simulink model "SimulationV2"  (R2016a)
settings: Solver=ode45  StartTime=0.0  StopTime=tfin  FixedStep=0.001  RelTol=1e-09
values from neighbouring files (symbols this model uses):
  ae0 = a2(1)    [Actionneurs.m]    (also in CoefficientsActionneurs.mat = 1.33983155374)
  ae1 = a2(2)    [Actionneurs.m]    (also in CoefficientsActionneurs.mat = 355.645740125)
  ae2 = a2(3)    [Actionneurs.m]    (also in CoefficientsActionneurs.mat = 1816.89307929)
  ae3 = a2(4)    [Actionneurs.m]    (also in CoefficientsActionneurs.mat = 704384.749782)
  as0 = a3(1)    [Actionneurs.m]    (also in CoefficientsActionneurs.mat = 0.0586667067)
  as1 = a3(2)    [Actionneurs.m]    (also in CoefficientsActionneurs.mat = 22.4105523392)
  as2 = a3(3)    [Actionneurs.m]    (also in CoefficientsActionneurs.mat = 860.394175869)
  as3 = a3(4)    [Actionneurs.m]    (also in CoefficientsActionneurs.mat = 233710.908706)
  be1 = 13.029359254409743    (= 13.0293592544)    [Actionneurs.m]    (also in CoefficientsActionneurs.mat)
  g = 9.81    [bancEssaiConstantes.m]    (also in trajectoire.m = sqrt(1 + (df).^2))
  Jx = 1169e-06    (= 0.001169)    [bancEssaiConstantes.m]
  Jy = Jx    (= 0.001169)    [bancEssaiConstantes.m]
  LA = LL    (= 0.115)    [bancEssaiConstantes.m]
  LB = LL    (= 0.115)    [bancEssaiConstantes.m]
  LC = LL    (= 0.115)    [bancEssaiConstantes.m]
  mS = 0.0080    (= 0.008)    [bancEssaiConstantes.m]
  mSeff = mS+JS/rS^2    (= 0.0112)    [bancEssaiConstantes.m]
  mtot = mP + sig*mS    [bancEssaiConstantes.m]
  Pzeq = .015    (= 0.015)    [run_bancessai.m]
  RA = RR    (= 3.6)    [bancEssaiConstantes.m]
  RB = RR    (= 3.6)    [bancEssaiConstantes.m]
  RC = RR    (= 3.6)    [bancEssaiConstantes.m]
  Vmax = 16.0    (= 16)    [bancEssaiConstantes.m]
  XA = +rABC    (= 0.0952)    [bancEssaiConstantes.m]
  XB = -rABC*sind(30)    [bancEssaiConstantes.m]
  XC = -rABC*sind(30)    [bancEssaiConstantes.m]
  XD = +rDEF*sind(30)    [bancEssaiConstantes.m]
  XE = -rDEF    (= -0.08)    [bancEssaiConstantes.m]
  XF = +rDEF*sind(30)    [bancEssaiConstantes.m]
  YA = 0.0    (= 0)    [bancEssaiConstantes.m]
  YB = +rABC*cosd(30)    [bancEssaiConstantes.m]
  YC = -rABC*cosd(30)    [bancEssaiConstantes.m]
  YD = +rDEF*cosd(30)    [bancEssaiConstantes.m]
  YE = 0.0    (= 0)    [bancEssaiConstantes.m]
  YF = -rDEF*cosd(30)    [bancEssaiConstantes.m]
settings Model: Creator=delafontaine  LastModifiedBy=Jaco_
settings SolverCC: AlgebraicLoopSolver=LineSearch
settings DataIOCC: LimitDataPoints=on  SaveFormat=Array  SignalLoggingSaveFormat=ModelDataLogs
settings DebuggingCC: UnderspecifiedInitializationDetection=Classic  MergeDetectMultiDrivingBlocksExec=none  MultiTaskDSMMsg=warning  MultiTaskCondExecSysMsg=none
settings HardwareCC: ProdBitPerPointer=32  ProdLargestAtomicFloat=None  ProdIntDivRoundTo=Undefined  ProdEndianess=Unspecified  ProdWordSize=32  ProdHWDeviceType=32-bit Generic
settings ModelReferenceCC: PropagateSignalLabelsOutOfModel=off
settings ConfigComp: CovModelRefEnable=Off  CovSFcnEnable=off

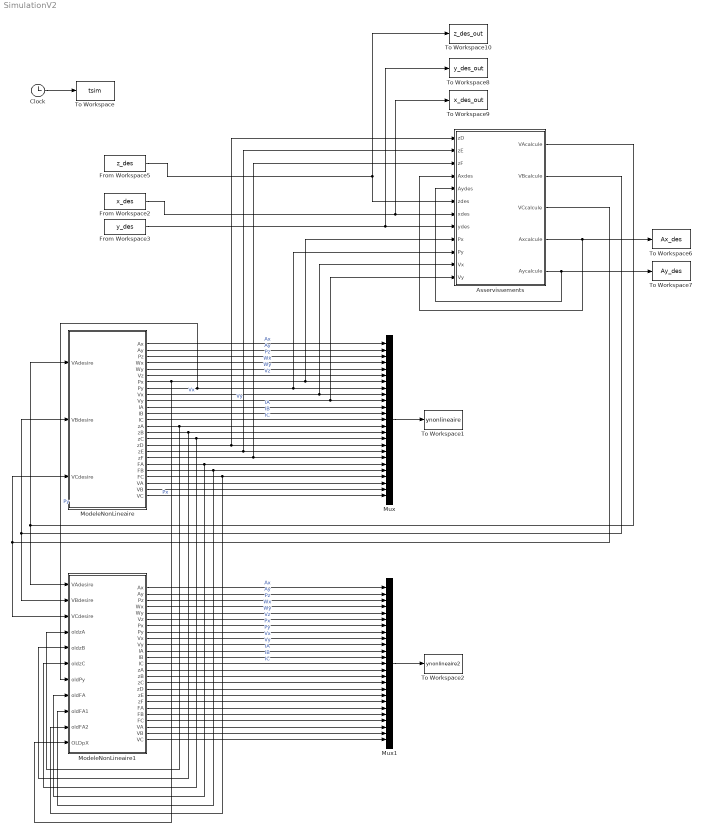
== system SimulationV2 ==
  Asservissements : Subsystem
      mask help: Simulink:masks:GenSFuncDesc_MD
      mask Help: eval('feval(''rtwprivate'',''rtwhelpview'',''rtw_sfcn_block'')');
  Clock : Clock
  From Workspace2 : FromWorkspace  VariableName=x_des  SampleTime=0  Interpolate=off  OutputAfterFinalValue=Holding final value
  From Workspace3 : FromWorkspace  VariableName=y_des  SampleTime=0  Interpolate=off  OutputAfterFinalValue=Holding final value
  From Workspace5 : FromWorkspace  VariableName=z_des  SampleTime=0  Interpolate=off  OutputAfterFinalValue=Holding final value
  ModeleNonLineaire : Subsystem
      mask help: Simulink:masks:GenSFuncDesc_MD
      mask Help: eval('feval(''rtwprivate'',''rtwhelpview'',''rtw_sfcn_block'')');
  ModeleNonLineaire1 : Subsystem
      mask help: Simulink:masks:GenSFuncDesc_MD
      mask Help: eval('feval(''rtwprivate'',''rtwhelpview'',''rtw_sfcn_block'')');
  Mux : Mux  Inputs=25
  Mux1 : Mux  Inputs=25
  To Workspace : ToWorkspace  VariableName=tsim  SampleTime=-1
  To Workspace1 : ToWorkspace  VariableName=ynonlineaire  SampleTime=-1
  To Workspace10 : ToWorkspace  VariableName=z_des_out  SampleTime=-1
  To Workspace2 : ToWorkspace  VariableName=ynonlineaire2  SampleTime=-1
  To Workspace6 : ToWorkspace  VariableName=Ax_des  SampleTime=-1
  To Workspace7 : ToWorkspace  VariableName=Ay_des  SampleTime=-1
  To Workspace8 : ToWorkspace  VariableName=y_des_out  SampleTime=-1
  To Workspace9 : ToWorkspace  VariableName=x_des_out  SampleTime=-1
  wires:
  Mux/1 -> To Workspace1/1
  Clock/1 -> To Workspace/1
  From Workspace5/1 -> Asservissements/6(zdes), To Workspace10/1
  ModeleNonLineaire/1(Ax) -> Mux/1  "Ax"
  ModeleNonLineaire/2(Ay) -> Mux/2  "Ay"
  ModeleNonLineaire/3(Pz) -> Mux/3  "Pz"
  ModeleNonLineaire/4(Wx) -> Mux/4  "Wx"
  ModeleNonLineaire/5(Wy) -> Mux/5  "Wy"
  ModeleNonLineaire/6(Vz) -> Mux/6  "Vz"
  ModeleNonLineaire/7(Px) -> ModeleNonLineaire1/11("OLDpX "), Asservissements/9(Px), Mux/7  "Px"
  ModeleNonLineaire/8(Py) -> ModeleNonLineaire1/7(oldPy), Asservissements/10(Py), Mux/8  "Py"
  ModeleNonLineaire/9(Vx) -> Asservissements/11(Vx), Mux/9  "Vx"
  ModeleNonLineaire/10(Vy) -> Asservissements/12(Vy), Mux/10  "Vy"
  ModeleNonLineaire/11(IA) -> Mux/11  "IA"
  ModeleNonLineaire/12(IB) -> Mux/12  "IB"
  ModeleNonLineaire/13(IC) -> Mux/13  "IC"
  From Workspace3/1 -> Asservissements/8(ydes), To Workspace8/1
  From Workspace2/1 -> Asservissements/7(xdes), To Workspace9/1
  ModeleNonLineaire/20(FA) -> ModeleNonLineaire1/8(oldFA), Mux/20
  ModeleNonLineaire/21(FB) -> ModeleNonLineaire1/9(oldFA1), Mux/21
  ModeleNonLineaire/22(FC) -> ModeleNonLineaire1/10(oldFA2), Mux/22
  ModeleNonLineaire/23(VA) -> Mux/23
  ModeleNonLineaire/24(VB) -> Mux/24
  ModeleNonLineaire/25(VC) -> Mux/25
  ModeleNonLineaire/17(zD) -> Asservissements/1(zD), Mux/17
  ModeleNonLineaire/18(zE) -> Asservissements/2(zE), Mux/18
  ModeleNonLineaire/19(zF) -> Asservissements/3(zF), Mux/19
  ModeleNonLineaire/14(zA) -> ModeleNonLineaire1/4(oldzA), Mux/14
  ModeleNonLineaire/15(zB) -> ModeleNonLineaire1/5(oldzB), Mux/15
  ModeleNonLineaire/16(zC) -> ModeleNonLineaire1/6(oldzC), Mux/16
  Asservissements/4(Axcalcule) -> Asservissements/4(Axdes), To Workspace6/1
  Asservissements/5(Aycalcule) -> Asservissements/5(Aydes), To Workspace7/1
  Mux1/1 -> To Workspace2/1
  ModeleNonLineaire1/1(Ax) -> Mux1/1  "Ax"
  ModeleNonLineaire1/2(Ay) -> Mux1/2  "Ay"
  ModeleNonLineaire1/3(Pz) -> Mux1/3  "Pz"
  ModeleNonLineaire1/4(Wx) -> Mux1/4  "Wx"
  ModeleNonLineaire1/5(Wy) -> Mux1/5  "Wy"
  ModeleNonLineaire1/6(Vz) -> Mux1/6  "Vz"
  ModeleNonLineaire1/7(Px) -> Mux1/7  "Px"
  ModeleNonLineaire1/8(Py) -> Mux1/8  "Py"
  ModeleNonLineaire1/9(Vx) -> Mux1/9  "Vx"
  ModeleNonLineaire1/10(Vy) -> Mux1/10  "Vy"
  ModeleNonLineaire1/11(IA) -> Mux1/11  "IA"
  ModeleNonLineaire1/12(IB) -> Mux1/12  "IB"
  ModeleNonLineaire1/13(IC) -> Mux1/13  "IC"
  ModeleNonLineaire1/20(FA) -> Mux1/20
  ModeleNonLineaire1/21(FB) -> Mux1/21
  ModeleNonLineaire1/22(FC) -> Mux1/22
  ModeleNonLineaire1/23(VA) -> Mux1/23
  ModeleNonLineaire1/24(VB) -> Mux1/24
  ModeleNonLineaire1/25(VC) -> Mux1/25
  ModeleNonLineaire1/17(zD) -> Mux1/17
  ModeleNonLineaire1/18(zE) -> Mux1/18
  ModeleNonLineaire1/19(zF) -> Mux1/19
  ModeleNonLineaire1/14(zA) -> Mux1/14
  ModeleNonLineaire1/15(zB) -> Mux1/15
  ModeleNonLineaire1/16(zC) -> Mux1/16
  Asservissements/1(VAcalcule) -> ModeleNonLineaire/1(VAdesire), ModeleNonLineaire1/1(VAdesire)
  Asservissements/2(VBcalcule) -> ModeleNonLineaire/2(VBdesire), ModeleNonLineaire1/2(VBdesire)
  Asservissements/3(VCcalcule) -> ModeleNonLineaire/3(VCdesire), ModeleNonLineaire1/3(VCdesire)

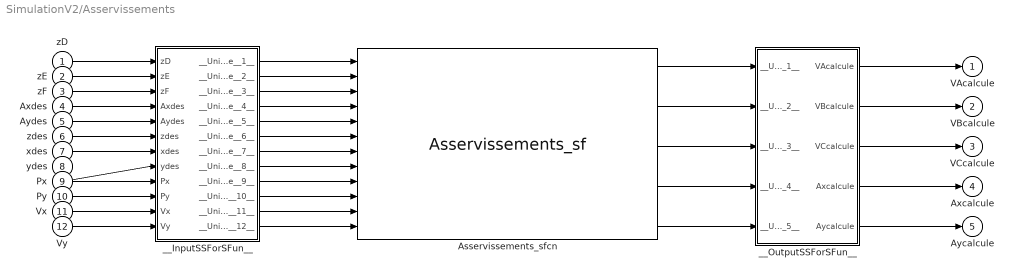
== system SimulationV2/Asservissements ==
  zD : Inport
  zE : Inport  Port=2
  zF : Inport  Port=3
  Axdes : Inport  Port=4
  Aydes : Inport  Port=5
  zdes : Inport  Port=6
  xdes : Inport  Port=7
  ydes : Inport  Port=8
  Px : Inport  Port=9
  Py : Inport  Port=10
  Vx : Inport  Port=11
  Vy : Inport  Port=12
  Asservissements_sfcn : S-Function  FunctionName=Asservissements_sf  SFunctionModules=""  SFunctionDeploymentMode=off  EnableBusSupport=off  mask{rtw_sf_name=Asservissements_sf, showVar=off}
      mask prompts: rtw_sf_name "Simulink:masks:GenSFuncName_MP"; showVar "Simulink:masks:GenSFuncShowModuleList_MP"
      mask help: Simulink:masks:GenSFuncDesc_MD
      mask init:
      | displist = '';
      | if ~strcmp(get_param(gcb, 'FunctionName'), rtw_sf_name);
      |   set_param(gcb, 'FunctionName', rtw_sf_name);
      | end
      | % Check if we are generating code
      | rtw_mode = false;
      | if strcmpi(get_param(bdroot(gcb),'SimulationStatus'),'Initializing')
      | 	rtw_mode = strcmpi(get_param(bdroot(gcb),'BuildingRTWCode'),'on') && ...
      | 		~strcmpi(get_param(bdroot(gcb),'TargetStyle'),'SimulationTarget');
      | end
      | if showVar || rtw_mode
      | 	if exist('rtwsfunc') == 2 | exist('rtwsfunc') == 6
      | 		tmplist = rtwsfunc(rtw_sf_name,gcb);
      | 		tmplist = DAStudio.message('Simulink:masks:GenSFuncListOfModules_IC', tmplist);
      | 	elseif showVar
      | 		tmplist1 = DAStudio.message('Simulink:masks:GenSFuncListOfModules_IC', '');
      |         tmplist2 = DAStudio.message('Simulink:masks:GenSFuncNotLicensed_IC');
      |         tmplist = [tmplist1 tmplist2];
      |  	end
      | end
      | if showVar
      |   displist = tmplist;
      | end
      settings: CopyFcn=|
      | if ~strcmp(get_param(gcb,'Linkstatus'),'none') && ...
      | ~strcmp(get_param(gcb,'Linkstatus'),'implicit')
      |   set_param(gcb,'LinkStatus','none');
      | end
      mask Help: eval('feval(''rtwprivate'',''rtwhelpview'',''rtw_sfcn_block'')');
      mask Display:
      | port_label('input',1,'zD');
      | port_label('input',2,'zE');
      | port_label('input',3,'zF');
      | port_label('input',4,'Axdes');
      | port_label('input',5,'Aydes');
      | port_label('input',6,'zdes');
      | port_label('input',7,'xdes');
      | port_label('input',8,'ydes');
      | port_label('input',9,'Px');
      | port_label('input',10,'Py');
      | port_label('input',11,'Vx');
      | port_label('input',12,'Vy');
      | port_label('output',1,'VAcalcule');
      | port_label('output',2,'VBcalcule');
      | port_label('output',3,'VCcalcule');
      | port_label('output',4,'Axcalcule');
      | port_label('output',5,'Aycalcule');
  __InputSSForSFun__ : Subsystem
  __OutputSSForSFun__ : Subsystem
  VAcalcule : Outport
  VBcalcule : Outport  Port=2
  VCcalcule : Outport  Port=3
  Axcalcule : Outport  Port=4
  Aycalcule : Outport  Port=5
  wires:
  zD/1 -> __InputSSForSFun__/1(zD)
  zE/1 -> __InputSSForSFun__/2(zE)
  zF/1 -> __InputSSForSFun__/3(zF)
  Axdes/1 -> __InputSSForSFun__/4(Axdes)
  Aydes/1 -> __InputSSForSFun__/5(Aydes)
  zdes/1 -> __InputSSForSFun__/6(zdes)
  xdes/1 -> __InputSSForSFun__/7(xdes)
  ydes/1 -> __InputSSForSFun__/8(ydes)
  Px/1 -> __InputSSForSFun__/9(Px)
  Py/1 -> __InputSSForSFun__/10(Py)
  Vx/1 -> __InputSSForSFun__/11(Vx)
  Vy/1 -> __InputSSForSFun__/12(Vy)
  __InputSSForSFun__/1(__UniqueOutportName__1__) -> Asservissements_sfcn/1
  __InputSSForSFun__/2(__UniqueOutportName__2__) -> Asservissements_sfcn/2
  __InputSSForSFun__/3(__UniqueOutportName__3__) -> Asservissements_sfcn/3
  __InputSSForSFun__/4(__UniqueOutportName__4__) -> Asservissements_sfcn/4
  __InputSSForSFun__/5(__UniqueOutportName__5__) -> Asservissements_sfcn/5
  __InputSSForSFun__/6(__UniqueOutportName__6__) -> Asservissements_sfcn/6
  __InputSSForSFun__/7(__UniqueOutportName__7__) -> Asservissements_sfcn/7
  __InputSSForSFun__/8(__UniqueOutportName__8__) -> Asservissements_sfcn/8
  __InputSSForSFun__/9(__UniqueOutportName__9__) -> Asservissements_sfcn/9
  __InputSSForSFun__/10(__UniqueOutportName__10__) -> Asservissements_sfcn/10
  __InputSSForSFun__/11(__UniqueOutportName__11__) -> Asservissements_sfcn/11
  __InputSSForSFun__/12(__UniqueOutportName__12__) -> Asservissements_sfcn/12
  Asservissements_sfcn/1 -> __OutputSSForSFun__/1(__UniqueInportName__1__)
  Asservissements_sfcn/2 -> __OutputSSForSFun__/2(__UniqueInportName__2__)
  Asservissements_sfcn/3 -> __OutputSSForSFun__/3(__UniqueInportName__3__)
  Asservissements_sfcn/4 -> __OutputSSForSFun__/4(__UniqueInportName__4__)
  Asservissements_sfcn/5 -> __OutputSSForSFun__/5(__UniqueInportName__5__)
  __OutputSSForSFun__/1(VAcalcule) -> VAcalcule/1
  __OutputSSForSFun__/2(VBcalcule) -> VBcalcule/1
  __OutputSSForSFun__/3(VCcalcule) -> VCcalcule/1
  __OutputSSForSFun__/4(Axcalcule) -> Axcalcule/1
  __OutputSSForSFun__/5(Aycalcule) -> Aycalcule/1

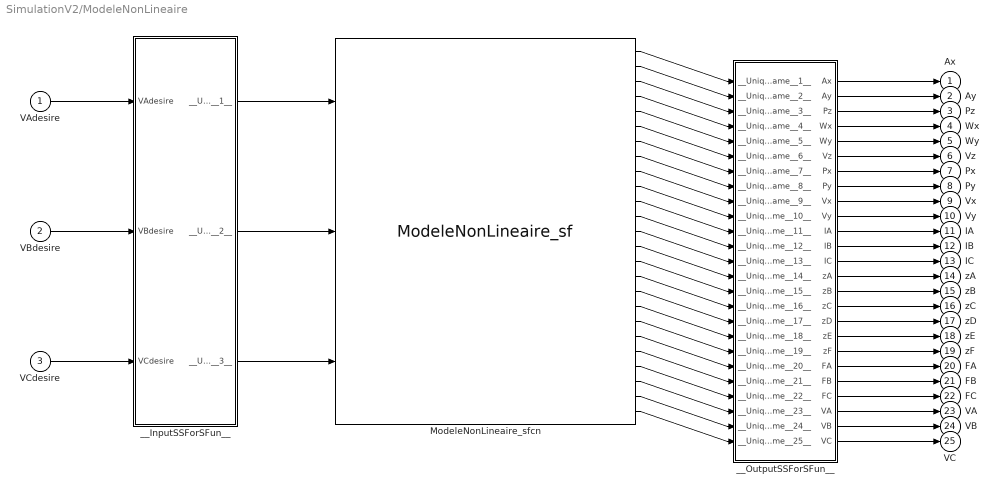
== system SimulationV2/ModeleNonLineaire ==
  VAdesire : Inport
  VBdesire : Inport  Port=2
  VCdesire : Inport  Port=3
  ModeleNonLineaire_sfcn : S-Function  FunctionName=ModeleNonLineaire_sf  SFunctionModules=""  SFunctionDeploymentMode=off  EnableBusSupport=off  mask{rtw_sf_name=ModeleNonLineaire_sf, showVar=off}
      mask prompts: rtw_sf_name "Simulink:masks:GenSFuncName_MP"; showVar "Simulink:masks:GenSFuncShowModuleList_MP"
      mask help: Simulink:masks:GenSFuncDesc_MD
      mask init: same as SimulationV2/Asservissements/Asservissements_sfcn
      settings: CopyFcn=|
      | if ~strcmp(get_param(gcb,'Linkstatus'),'none') && ...
      | ~strcmp(get_param(gcb,'Linkstatus'),'implicit')
      |   set_param(gcb,'LinkStatus','none');
      | end
      mask Help: eval('feval(''rtwprivate'',''rtwhelpview'',''rtw_sfcn_block'')');
      mask Display:
      | port_label('input',1,'VAdesire');
      | port_label('input',2,'VBdesire');
      | port_label('input',3,'VCdesire');
      | port_label('output',1,'Ax');
      | port_label('output',2,'Ay');
      | port_label('output',3,'Pz');
      | port_label('output',4,'Wx');
      | port_label('output',5,'Wy');
      | port_label('output',6,'Vz');
      | port_label('output',7,'Px');
      | port_label('output',8,'Py');
      | port_label('output',9,'Vx');
      | port_label('output',10,'Vy');
      | port_label('output',11,'IA');
      | port_label('output',12,'IB');
      | port_label('output',13,'IC');
      | port_label('output',14,'zA');
      | port_label('output',15,'zB');
      | port_label('output',16,'zC');
      | port_label('output',17,'zD');
      | port_label('output',18,'zE');
      | port_label('output',19,'zF');
      | port_label('output',20,'FA');
      | port_label('output',21,'FB');
      | port_label('output',22,'FC');
      | port_label('output',23,'VA');
      | port_label('output',24,'VB');
      | port_label('output',25,'VC');
  __InputSSForSFun__ : Subsystem
  __OutputSSForSFun__ : Subsystem
  Ax : Outport
  Ay : Outport  Port=2
  Pz : Outport  Port=3
  Wx : Outport  Port=4
  Wy : Outport  Port=5
  Vz : Outport  Port=6
  Px : Outport  Port=7
  Py : Outport  Port=8
  Vx : Outport  Port=9
  Vy : Outport  Port=10
  IA : Outport  Port=11
  IB : Outport  Port=12
  IC : Outport  Port=13
  zA : Outport  Port=14
  zB : Outport  Port=15
  zC : Outport  Port=16
  zD : Outport  Port=17
  zE : Outport  Port=18
  zF : Outport  Port=19
  FA : Outport  Port=20
  FB : Outport  Port=21
  FC : Outport  Port=22
  VA : Outport  Port=23
  VB : Outport  Port=24
  VC : Outport  Port=25
  wires:
  VAdesire/1 -> __InputSSForSFun__/1(VAdesire)
  VBdesire/1 -> __InputSSForSFun__/2(VBdesire)
  VCdesire/1 -> __InputSSForSFun__/3(VCdesire)
  __InputSSForSFun__/1(__UniqueOutportName__1__) -> ModeleNonLineaire_sfcn/1
  __InputSSForSFun__/2(__UniqueOutportName__2__) -> ModeleNonLineaire_sfcn/2
  __InputSSForSFun__/3(__UniqueOutportName__3__) -> ModeleNonLineaire_sfcn/3
  ModeleNonLineaire_sfcn/1 -> __OutputSSForSFun__/1(__UniqueInportName__1__)
  ModeleNonLineaire_sfcn/2 -> __OutputSSForSFun__/2(__UniqueInportName__2__)
  ModeleNonLineaire_sfcn/3 -> __OutputSSForSFun__/3(__UniqueInportName__3__)
  ModeleNonLineaire_sfcn/4 -> __OutputSSForSFun__/4(__UniqueInportName__4__)
  ModeleNonLineaire_sfcn/5 -> __OutputSSForSFun__/5(__UniqueInportName__5__)
  ModeleNonLineaire_sfcn/6 -> __OutputSSForSFun__/6(__UniqueInportName__6__)
  ModeleNonLineaire_sfcn/7 -> __OutputSSForSFun__/7(__UniqueInportName__7__)
  ModeleNonLineaire_sfcn/8 -> __OutputSSForSFun__/8(__UniqueInportName__8__)
  ModeleNonLineaire_sfcn/9 -> __OutputSSForSFun__/9(__UniqueInportName__9__)
  ModeleNonLineaire_sfcn/10 -> __OutputSSForSFun__/10(__UniqueInportName__10__)
  ModeleNonLineaire_sfcn/11 -> __OutputSSForSFun__/11(__UniqueInportName__11__)
  ModeleNonLineaire_sfcn/12 -> __OutputSSForSFun__/12(__UniqueInportName__12__)
  ModeleNonLineaire_sfcn/13 -> __OutputSSForSFun__/13(__UniqueInportName__13__)
  ModeleNonLineaire_sfcn/14 -> __OutputSSForSFun__/14(__UniqueInportName__14__)
  ModeleNonLineaire_sfcn/15 -> __OutputSSForSFun__/15(__UniqueInportName__15__)
  ModeleNonLineaire_sfcn/16 -> __OutputSSForSFun__/16(__UniqueInportName__16__)
  ModeleNonLineaire_sfcn/17 -> __OutputSSForSFun__/17(__UniqueInportName__17__)
  ModeleNonLineaire_sfcn/18 -> __OutputSSForSFun__/18(__UniqueInportName__18__)
  ModeleNonLineaire_sfcn/19 -> __OutputSSForSFun__/19(__UniqueInportName__19__)
  ModeleNonLineaire_sfcn/20 -> __OutputSSForSFun__/20(__UniqueInportName__20__)
  ModeleNonLineaire_sfcn/21 -> __OutputSSForSFun__/21(__UniqueInportName__21__)
  ModeleNonLineaire_sfcn/22 -> __OutputSSForSFun__/22(__UniqueInportName__22__)
  ModeleNonLineaire_sfcn/23 -> __OutputSSForSFun__/23(__UniqueInportName__23__)
  ModeleNonLineaire_sfcn/24 -> __OutputSSForSFun__/24(__UniqueInportName__24__)
  ModeleNonLineaire_sfcn/25 -> __OutputSSForSFun__/25(__UniqueInportName__25__)
  __OutputSSForSFun__/1(Ax) -> Ax/1
  __OutputSSForSFun__/2(Ay) -> Ay/1
  __OutputSSForSFun__/3(Pz) -> Pz/1
  __OutputSSForSFun__/4(Wx) -> Wx/1
  __OutputSSForSFun__/5(Wy) -> Wy/1
  __OutputSSForSFun__/6(Vz) -> Vz/1
  __OutputSSForSFun__/7(Px) -> Px/1
  __OutputSSForSFun__/8(Py) -> Py/1
  __OutputSSForSFun__/9(Vx) -> Vx/1
  __OutputSSForSFun__/10(Vy) -> Vy/1
  __OutputSSForSFun__/11(IA) -> IA/1
  __OutputSSForSFun__/12(IB) -> IB/1
  __OutputSSForSFun__/13(IC) -> IC/1
  __OutputSSForSFun__/14(zA) -> zA/1
  __OutputSSForSFun__/15(zB) -> zB/1
  __OutputSSForSFun__/16(zC) -> zC/1
  __OutputSSForSFun__/17(zD) -> zD/1
  __OutputSSForSFun__/18(zE) -> zE/1
  __OutputSSForSFun__/19(zF) -> zF/1
  __OutputSSForSFun__/20(FA) -> FA/1
  __OutputSSForSFun__/21(FB) -> FB/1
  __OutputSSForSFun__/22(FC) -> FC/1
  __OutputSSForSFun__/23(VA) -> VA/1
  __OutputSSForSFun__/24(VB) -> VB/1
  __OutputSSForSFun__/25(VC) -> VC/1

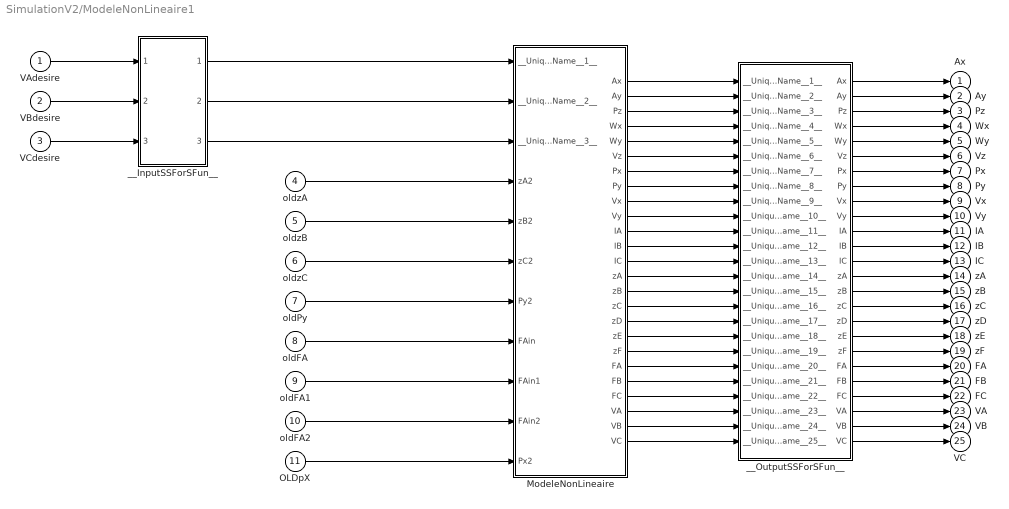
== system SimulationV2/ModeleNonLineaire1 ==
  VAdesire : Inport
  VBdesire : Inport  Port=2
  VCdesire : Inport  Port=3
  oldzA : Inport  Port=4
  oldzB : Inport  Port=5
  oldzC : Inport  Port=6
  oldPy : Inport  Port=7
  oldFA : Inport  Port=8
  oldFA1 : Inport  Port=9
  oldFA2 : Inport  Port=10
  "OLDpX " : Inport  Port=11
  ModeleNonLineaire : Subsystem
  __InputSSForSFun__ : Subsystem
  __OutputSSForSFun__ : Subsystem
  Ax : Outport
  Ay : Outport  Port=2
  Pz : Outport  Port=3
  Wx : Outport  Port=4
  Wy : Outport  Port=5
  Vz : Outport  Port=6
  Px : Outport  Port=7
  Py : Outport  Port=8
  Vx : Outport  Port=9
  Vy : Outport  Port=10
  IA : Outport  Port=11
  IB : Outport  Port=12
  IC : Outport  Port=13
  zA : Outport  Port=14
  zB : Outport  Port=15
  zC : Outport  Port=16
  zD : Outport  Port=17
  zE : Outport  Port=18
  zF : Outport  Port=19
  FA : Outport  Port=20
  FB : Outport  Port=21
  FC : Outport  Port=22
  VA : Outport  Port=23
  VB : Outport  Port=24
  VC : Outport  Port=25
  wires:
  VAdesire/1 -> __InputSSForSFun__/1(VAdesire)
  VBdesire/1 -> __InputSSForSFun__/2(VBdesire)
  VCdesire/1 -> __InputSSForSFun__/3(VCdesire)
  __InputSSForSFun__/1(__UniqueOutportName__1__) -> ModeleNonLineaire/1(__UniqueInportName__1__)
  __InputSSForSFun__/2(__UniqueOutportName__2__) -> ModeleNonLineaire/2(__UniqueInportName__2__)
  __InputSSForSFun__/3(__UniqueOutportName__3__) -> ModeleNonLineaire/3(__UniqueInportName__3__)
  __OutputSSForSFun__/1(Ax) -> Ax/1
  __OutputSSForSFun__/2(Ay) -> Ay/1
  __OutputSSForSFun__/3(Pz) -> Pz/1
  __OutputSSForSFun__/4(Wx) -> Wx/1
  __OutputSSForSFun__/5(Wy) -> Wy/1
  __OutputSSForSFun__/6(Vz) -> Vz/1
  __OutputSSForSFun__/7(Px) -> Px/1
  __OutputSSForSFun__/8(Py) -> Py/1
  __OutputSSForSFun__/9(Vx) -> Vx/1
  __OutputSSForSFun__/10(Vy) -> Vy/1
  __OutputSSForSFun__/11(IA) -> IA/1
  __OutputSSForSFun__/12(IB) -> IB/1
  __OutputSSForSFun__/13(IC) -> IC/1
  __OutputSSForSFun__/14(zA) -> zA/1
  __OutputSSForSFun__/15(zB) -> zB/1
  __OutputSSForSFun__/16(zC) -> zC/1
  __OutputSSForSFun__/17(zD) -> zD/1
  __OutputSSForSFun__/18(zE) -> zE/1
  __OutputSSForSFun__/19(zF) -> zF/1
  __OutputSSForSFun__/20(FA) -> FA/1
  __OutputSSForSFun__/21(FB) -> FB/1
  __OutputSSForSFun__/22(FC) -> FC/1
  __OutputSSForSFun__/23(VA) -> VA/1
  __OutputSSForSFun__/24(VB) -> VB/1
  __OutputSSForSFun__/25(VC) -> VC/1
  ModeleNonLineaire/23(VA) -> __OutputSSForSFun__/23(__UniqueInportName__23__)
  ModeleNonLineaire/24(VB) -> __OutputSSForSFun__/24(__UniqueInportName__24__)
  ModeleNonLineaire/25(VC) -> __OutputSSForSFun__/25(__UniqueInportName__25__)
  ModeleNonLineaire/11(IA) -> __OutputSSForSFun__/11(__UniqueInportName__11__)
  ModeleNonLineaire/12(IB) -> __OutputSSForSFun__/12(__UniqueInportName__12__)
  ModeleNonLineaire/13(IC) -> __OutputSSForSFun__/13(__UniqueInportName__13__)
  ModeleNonLineaire/20(FA) -> __OutputSSForSFun__/20(__UniqueInportName__20__)
  ModeleNonLineaire/21(FB) -> __OutputSSForSFun__/21(__UniqueInportName__21__)
  ModeleNonLineaire/22(FC) -> __OutputSSForSFun__/22(__UniqueInportName__22__)
  oldzA/1 -> ModeleNonLineaire/4(zA2)
  oldzB/1 -> ModeleNonLineaire/5(zB2)
  oldzC/1 -> ModeleNonLineaire/6(zC2)
  ModeleNonLineaire/6(Vz) -> __OutputSSForSFun__/6(__UniqueInportName__6__)
  oldPy/1 -> ModeleNonLineaire/7(Py2)
  ModeleNonLineaire/4(Wx) -> __OutputSSForSFun__/4(__UniqueInportName__4__)
  oldFA/1 -> ModeleNonLineaire/8(FAin)
  oldFA1/1 -> ModeleNonLineaire/9(FAin1)
  oldFA2/1 -> ModeleNonLineaire/10(FAin2)
  "OLDpX "/1 -> ModeleNonLineaire/11(Px2)
  ModeleNonLineaire/5(Wy) -> __OutputSSForSFun__/5(__UniqueInportName__5__)
  ModeleNonLineaire/1(Ax) -> __OutputSSForSFun__/1(__UniqueInportName__1__)
  ModeleNonLineaire/2(Ay) -> __OutputSSForSFun__/2(__UniqueInportName__2__)
  ModeleNonLineaire/14(zA) -> __OutputSSForSFun__/14(__UniqueInportName__14__)
  ModeleNonLineaire/15(zB) -> __OutputSSForSFun__/15(__UniqueInportName__15__)
  ModeleNonLineaire/16(zC) -> __OutputSSForSFun__/16(__UniqueInportName__16__)
  ModeleNonLineaire/17(zD) -> __OutputSSForSFun__/17(__UniqueInportName__17__)
  ModeleNonLineaire/18(zE) -> __OutputSSForSFun__/18(__UniqueInportName__18__)
  ModeleNonLineaire/19(zF) -> __OutputSSForSFun__/19(__UniqueInportName__19__)
  ModeleNonLineaire/3(Pz) -> __OutputSSForSFun__/3(__UniqueInportName__3__)
  ModeleNonLineaire/10(Vy) -> __OutputSSForSFun__/10(__UniqueInportName__10__)
  ModeleNonLineaire/9(Vx) -> __OutputSSForSFun__/9(__UniqueInportName__9__)
  ModeleNonLineaire/8(Py) -> __OutputSSForSFun__/8(__UniqueInportName__8__)
  ModeleNonLineaire/7(Px) -> __OutputSSForSFun__/7(__UniqueInportName__7__)

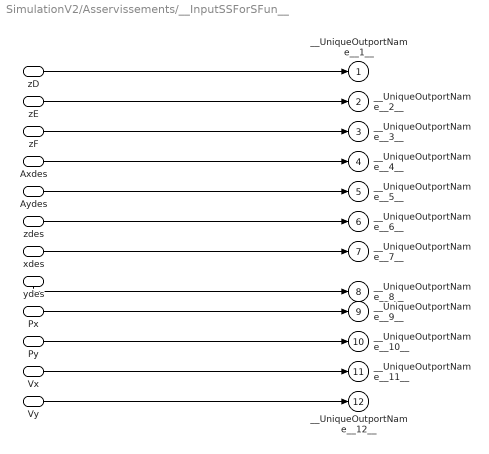
== system SimulationV2/Asservissements/__InputSSForSFun__ ==
  zD : Inport
  zE : Inport  Port=2
  zF : Inport  Port=3
  Axdes : Inport  Port=4
  Aydes : Inport  Port=5
  zdes : Inport  Port=6
  xdes : Inport  Port=7
  ydes : Inport  Port=8
  Px : Inport  Port=9
  Py : Inport  Port=10
  Vx : Inport  Port=11
  Vy : Inport  Port=12
  __UniqueOutportName__1__ : Outport
  __UniqueOutportName__2__ : Outport  Port=2
  __UniqueOutportName__3__ : Outport  Port=3
  __UniqueOutportName__4__ : Outport  Port=4
  __UniqueOutportName__5__ : Outport  Port=5
  __UniqueOutportName__6__ : Outport  Port=6
  __UniqueOutportName__7__ : Outport  Port=7
  __UniqueOutportName__8__ : Outport  Port=8
  __UniqueOutportName__9__ : Outport  Port=9
  __UniqueOutportName__10__ : Outport  Port=10
  __UniqueOutportName__11__ : Outport  Port=11
  __UniqueOutportName__12__ : Outport  Port=12
  wires:
  zD/1 -> __UniqueOutportName__1__/1
  zE/1 -> __UniqueOutportName__2__/1
  zF/1 -> __UniqueOutportName__3__/1
  Axdes/1 -> __UniqueOutportName__4__/1
  Aydes/1 -> __UniqueOutportName__5__/1
  zdes/1 -> __UniqueOutportName__6__/1
  xdes/1 -> __UniqueOutportName__7__/1
  ydes/1 -> __UniqueOutportName__8__/1
  Px/1 -> __UniqueOutportName__9__/1
  Py/1 -> __UniqueOutportName__10__/1
  Vx/1 -> __UniqueOutportName__11__/1
  Vy/1 -> __UniqueOutportName__12__/1

== system SimulationV2/Asservissements/__OutputSSForSFun__ ==
  __UniqueInportName__1__ : Inport
  __UniqueInportName__2__ : Inport  Port=2
  __UniqueInportName__3__ : Inport  Port=3
  __UniqueInportName__4__ : Inport  Port=4
  __UniqueInportName__5__ : Inport  Port=5
  VAcalcule : Outport
  VBcalcule : Outport  Port=2
  VCcalcule : Outport  Port=3
  Axcalcule : Outport  Port=4
  Aycalcule : Outport  Port=5
  wires:
  __UniqueInportName__1__/1 -> VAcalcule/1
  __UniqueInportName__2__/1 -> VBcalcule/1
  __UniqueInportName__3__/1 -> VCcalcule/1
  __UniqueInportName__4__/1 -> Axcalcule/1  "Ax_des"
  __UniqueInportName__5__/1 -> Aycalcule/1  "Ay_des"

== system SimulationV2/ModeleNonLineaire/__InputSSForSFun__ ==
  VAdesire : Inport
  VBdesire : Inport  Port=2
  VCdesire : Inport  Port=3
  __UniqueOutportName__1__ : Outport
  __UniqueOutportName__2__ : Outport  Port=2
  __UniqueOutportName__3__ : Outport  Port=3
  wires:
  VAdesire/1 -> __UniqueOutportName__1__/1
  VBdesire/1 -> __UniqueOutportName__2__/1
  VCdesire/1 -> __UniqueOutportName__3__/1

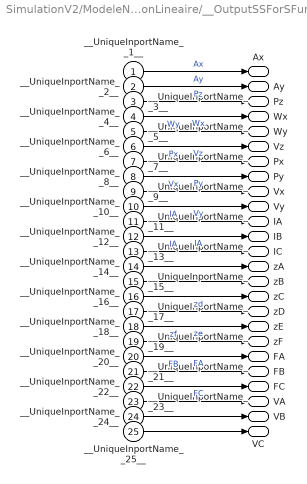
== system SimulationV2/ModeleNonLineaire/__OutputSSForSFun__ ==
  __UniqueInportName__1__ : Inport
  __UniqueInportName__2__ : Inport  Port=2
  __UniqueInportName__3__ : Inport  Port=3
  __UniqueInportName__4__ : Inport  Port=4
  __UniqueInportName__5__ : Inport  Port=5
  __UniqueInportName__6__ : Inport  Port=6
  __UniqueInportName__7__ : Inport  Port=7
  __UniqueInportName__8__ : Inport  Port=8
  __UniqueInportName__9__ : Inport  Port=9
  __UniqueInportName__10__ : Inport  Port=10
  __UniqueInportName__11__ : Inport  Port=11
  __UniqueInportName__12__ : Inport  Port=12
  __UniqueInportName__13__ : Inport  Port=13
  __UniqueInportName__14__ : Inport  Port=14
  __UniqueInportName__15__ : Inport  Port=15
  __UniqueInportName__16__ : Inport  Port=16
  __UniqueInportName__17__ : Inport  Port=17
  __UniqueInportName__18__ : Inport  Port=18
  __UniqueInportName__19__ : Inport  Port=19
  __UniqueInportName__20__ : Inport  Port=20
  __UniqueInportName__21__ : Inport  Port=21
  __UniqueInportName__22__ : Inport  Port=22
  __UniqueInportName__23__ : Inport  Port=23
  __UniqueInportName__24__ : Inport  Port=24
  __UniqueInportName__25__ : Inport  Port=25
  Ax : Outport
  Ay : Outport  Port=2
  Pz : Outport  Port=3
  Wx : Outport  Port=4
  Wy : Outport  Port=5
  Vz : Outport  Port=6
  Px : Outport  Port=7
  Py : Outport  Port=8
  Vx : Outport  Port=9
  Vy : Outport  Port=10
  IA : Outport  Port=11
  IB : Outport  Port=12
  IC : Outport  Port=13
  zA : Outport  Port=14
  zB : Outport  Port=15
  zC : Outport  Port=16
  zD : Outport  Port=17
  zE : Outport  Port=18
  zF : Outport  Port=19
  FA : Outport  Port=20
  FB : Outport  Port=21
  FC : Outport  Port=22
  VA : Outport  Port=23
  VB : Outport  Port=24
  VC : Outport  Port=25
  wires:
  __UniqueInportName__1__/1 -> Ax/1  "Ax"
  __UniqueInportName__2__/1 -> Ay/1  "Ay"
  __UniqueInportName__3__/1 -> Pz/1  "Pz"
  __UniqueInportName__4__/1 -> Wx/1  "Wx"
  __UniqueInportName__5__/1 -> Wy/1  "Wy"
  __UniqueInportName__6__/1 -> Vz/1  "Vz"
  __UniqueInportName__7__/1 -> Px/1  "Px"
  __UniqueInportName__8__/1 -> Py/1  "Py"
  __UniqueInportName__9__/1 -> Vx/1  "Vx"
  __UniqueInportName__10__/1 -> Vy/1  "Vy"
  __UniqueInportName__11__/1 -> IA/1  "IA"
  __UniqueInportName__12__/1 -> IB/1  "IA"
  __UniqueInportName__13__/1 -> IC/1  "IA"
  __UniqueInportName__14__/1 -> zA/1
  __UniqueInportName__15__/1 -> zB/1
  __UniqueInportName__16__/1 -> zC/1
  __UniqueInportName__17__/1 -> zD/1  "zd"
  __UniqueInportName__18__/1 -> zE/1  "ze"
  __UniqueInportName__19__/1 -> zF/1  "zf"
  __UniqueInportName__20__/1 -> FA/1  "FA"
  __UniqueInportName__21__/1 -> FB/1  "FB"
  __UniqueInportName__22__/1 -> FC/1  "FC"
  __UniqueInportName__23__/1 -> VA/1
  __UniqueInportName__24__/1 -> VB/1
  __UniqueInportName__25__/1 -> VC/1

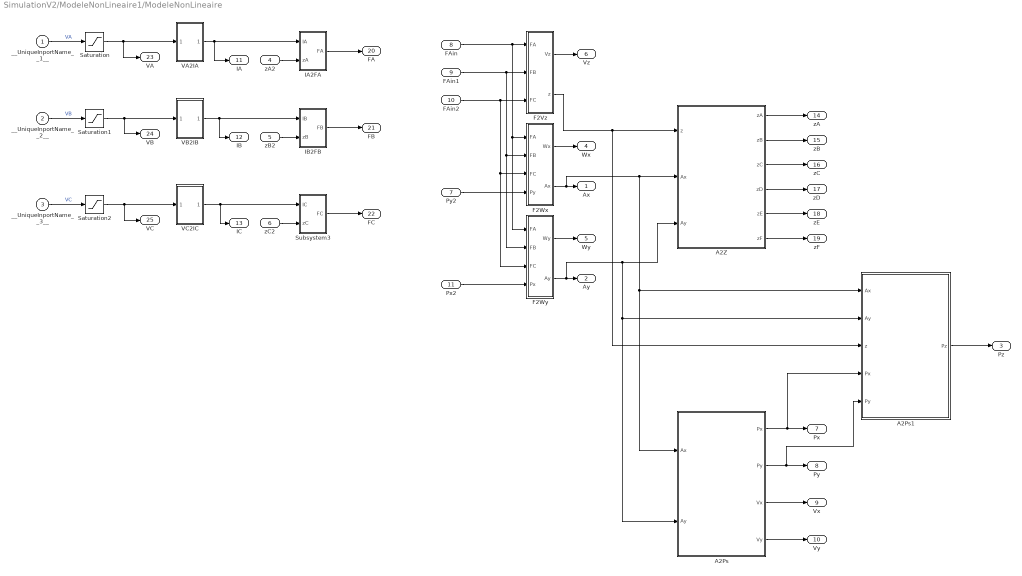
== system SimulationV2/ModeleNonLineaire1/ModeleNonLineaire ==
  __UniqueInportName__1__ : Inport
  __UniqueInportName__2__ : Inport  Port=2
  __UniqueInportName__3__ : Inport  Port=3
  zA2 : Inport  Port=4
  zB2 : Inport  Port=5
  zC2 : Inport  Port=6
  Py2 : Inport  Port=7
  FAin : Inport  Port=8
  FAin1 : Inport  Port=9
  FAin2 : Inport  Port=10
  Px2 : Inport  Port=11
  A2Ps : Subsystem
  A2Ps1 : Subsystem
  A2Z : Subsystem
  F2Vz : Subsystem
  F2Wx : Subsystem
  F2Wy : Subsystem
  IA2FA : Subsystem
  IB2FB : Subsystem
  Saturation : Saturate  UpperLimit=Vmax  LowerLimit=-Vmax
  Saturation1 : Saturate  UpperLimit=Vmax  LowerLimit=-Vmax
  Saturation2 : Saturate  UpperLimit=Vmax  LowerLimit=-Vmax
  Subsystem3 : Subsystem
  VA2IA : Subsystem
  VB2IB : Subsystem
  VC2IC : Subsystem
  Ax : Outport
  Ay : Outport  Port=2
  Pz : Outport  Port=3
  Wx : Outport  Port=4
  Wy : Outport  Port=5
  Vz : Outport  Port=6
  Px : Outport  Port=7
  Py : Outport  Port=8
  Vx : Outport  Port=9
  Vy : Outport  Port=10
  IA : Outport  Port=11
  IB : Outport  Port=12
  IC : Outport  Port=13
  zA : Outport  Port=14
  zB : Outport  Port=15
  zC : Outport  Port=16
  zD : Outport  Port=17
  zE : Outport  Port=18
  zF : Outport  Port=19
  FA : Outport  Port=20
  FB : Outport  Port=21
  FC : Outport  Port=22
  VA : Outport  Port=23
  VB : Outport  Port=24
  VC : Outport  Port=25
  wires:
  __UniqueInportName__1__/1 -> Saturation/1  "VA"
  __UniqueInportName__2__/1 -> Saturation1/1  "VB"
  __UniqueInportName__3__/1 -> Saturation2/1  "VC"
  Saturation/1 -> VA2IA/1(In1), VA/1
  VA2IA/1(Out1) -> IA2FA/1(IA), IA/1
  Saturation1/1 -> VB2IB/1(In1), VB/1
  VB2IB/1(Out1) -> IB/1, IB2FB/1(IB)
  Saturation2/1 -> VC2IC/1(In1), VC/1
  VC2IC/1(Out1) -> Subsystem3/1(IC), IC/1
  zA2/1 -> IA2FA/2(zA)
  IB2FB/1(FB) -> FB/1
  zB2/1 -> IB2FB/2(zB)
  IA2FA/1(FA) -> FA/1
  F2Vz/1(Vz) -> Vz/1
  Subsystem3/1(FC) -> FC/1
  Py2/1 -> F2Wx/4(Py)
  F2Wx/1(Wx) -> Wx/1
  Px2/1 -> F2Wy/4(Px)
  F2Wy/1(Wy) -> Wy/1
  FAin/1 -> F2Wy/1(FA), F2Wx/1(FA), F2Vz/1(FA)
  FAin2/1 -> F2Wy/3(FC), F2Wx/3(FC), F2Vz/3(FC)
  FAin1/1 -> F2Wy/2(FB), F2Wx/2(FB), F2Vz/2(FB)
  F2Wy/2(Ay) -> A2Ps/2(Ay), A2Ps1/2(Ay), A2Z/3(Ay), Ay/1
  F2Vz/2(z) -> A2Ps1/3(z), A2Z/1(z)
  F2Wx/2(Ax) -> A2Ps1/1(Ax), A2Ps/1(Ax), A2Z/2(Ax), Ax/1
  A2Z/1(zA) -> zA/1
  A2Z/2(zB) -> zB/1
  A2Z/3(zC) -> zC/1
  A2Z/4(zD) -> zD/1
  A2Z/5(zE) -> zE/1
  A2Z/6(zF) -> zF/1
  A2Ps/1(Px) -> A2Ps1/4(Px), Px/1
  A2Ps/2(Py) -> A2Ps1/5(Py), Py/1
  A2Ps/3(Vx) -> Vx/1
  A2Ps/4(Vy) -> Vy/1
  A2Ps1/1(Pz) -> Pz/1
  zC2/1 -> Subsystem3/2(zC)

== system SimulationV2/ModeleNonLineaire1/__InputSSForSFun__ ==
  VAdesire : Inport
  VBdesire : Inport  Port=2
  VCdesire : Inport  Port=3
  __UniqueOutportName__1__ : Outport
  __UniqueOutportName__2__ : Outport  Port=2
  __UniqueOutportName__3__ : Outport  Port=3
  wires:
  VAdesire/1 -> __UniqueOutportName__1__/1
  VBdesire/1 -> __UniqueOutportName__2__/1
  VCdesire/1 -> __UniqueOutportName__3__/1

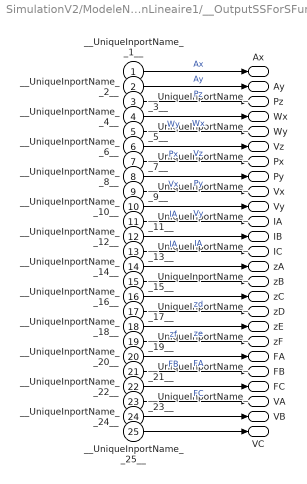
== system SimulationV2/ModeleNonLineaire1/__OutputSSForSFun__ ==
  __UniqueInportName__1__ : Inport
  __UniqueInportName__2__ : Inport  Port=2
  __UniqueInportName__3__ : Inport  Port=3
  __UniqueInportName__4__ : Inport  Port=4
  __UniqueInportName__5__ : Inport  Port=5
  __UniqueInportName__6__ : Inport  Port=6
  __UniqueInportName__7__ : Inport  Port=7
  __UniqueInportName__8__ : Inport  Port=8
  __UniqueInportName__9__ : Inport  Port=9
  __UniqueInportName__10__ : Inport  Port=10
  __UniqueInportName__11__ : Inport  Port=11
  __UniqueInportName__12__ : Inport  Port=12
  __UniqueInportName__13__ : Inport  Port=13
  __UniqueInportName__14__ : Inport  Port=14
  __UniqueInportName__15__ : Inport  Port=15
  __UniqueInportName__16__ : Inport  Port=16
  __UniqueInportName__17__ : Inport  Port=17
  __UniqueInportName__18__ : Inport  Port=18
  __UniqueInportName__19__ : Inport  Port=19
  __UniqueInportName__20__ : Inport  Port=20
  __UniqueInportName__21__ : Inport  Port=21
  __UniqueInportName__22__ : Inport  Port=22
  __UniqueInportName__23__ : Inport  Port=23
  __UniqueInportName__24__ : Inport  Port=24
  __UniqueInportName__25__ : Inport  Port=25
  Ax : Outport
  Ay : Outport  Port=2
  Pz : Outport  Port=3
  Wx : Outport  Port=4
  Wy : Outport  Port=5
  Vz : Outport  Port=6
  Px : Outport  Port=7
  Py : Outport  Port=8
  Vx : Outport  Port=9
  Vy : Outport  Port=10
  IA : Outport  Port=11
  IB : Outport  Port=12
  IC : Outport  Port=13
  zA : Outport  Port=14
  zB : Outport  Port=15
  zC : Outport  Port=16
  zD : Outport  Port=17
  zE : Outport  Port=18
  zF : Outport  Port=19
  FA : Outport  Port=20
  FB : Outport  Port=21
  FC : Outport  Port=22
  VA : Outport  Port=23
  VB : Outport  Port=24
  VC : Outport  Port=25
  wires:
  __UniqueInportName__1__/1 -> Ax/1  "Ax"
  __UniqueInportName__2__/1 -> Ay/1  "Ay"
  __UniqueInportName__3__/1 -> Pz/1  "Pz"
  __UniqueInportName__4__/1 -> Wx/1  "Wx"
  __UniqueInportName__5__/1 -> Wy/1  "Wy"
  __UniqueInportName__6__/1 -> Vz/1  "Vz"
  __UniqueInportName__7__/1 -> Px/1  "Px"
  __UniqueInportName__8__/1 -> Py/1  "Py"
  __UniqueInportName__9__/1 -> Vx/1  "Vx"
  __UniqueInportName__10__/1 -> Vy/1  "Vy"
  __UniqueInportName__11__/1 -> IA/1  "IA"
  __UniqueInportName__12__/1 -> IB/1  "IA"
  __UniqueInportName__13__/1 -> IC/1  "IA"
  __UniqueInportName__14__/1 -> zA/1
  __UniqueInportName__15__/1 -> zB/1
  __UniqueInportName__16__/1 -> zC/1
  __UniqueInportName__17__/1 -> zD/1  "zd"
  __UniqueInportName__18__/1 -> zE/1  "ze"
  __UniqueInportName__19__/1 -> zF/1  "zf"
  __UniqueInportName__20__/1 -> FA/1  "FA"
  __UniqueInportName__21__/1 -> FB/1  "FB"
  __UniqueInportName__22__/1 -> FC/1  "FC"
  __UniqueInportName__23__/1 -> VA/1
  __UniqueInportName__24__/1 -> VB/1
  __UniqueInportName__25__/1 -> VC/1

== system SimulationV2/ModeleNonLineaire1/ModeleNonLineaire/A2Ps ==
  Ax : Inport
  Ay : Inport  Port=2
  Gain : Gain  Gain=mS*g/mSeff
  Gain1 : Gain  Gain=-mS*g/mSeff
  Integrator{,1..3} (4 alike) : Integrator
  Px : Outport
  Py : Outport  Port=2
  Vx : Outport  Port=3
  Vy : Outport  Port=4
  wires:
  Ax/1 -> Gain/1
  Ay/1 -> Gain1/1
  Gain/1 -> Integrator/1
  Gain1/1 -> Integrator1/1
  Integrator1/1 -> Vx/1, Integrator3/1
  Integrator/1 -> Vy/1, Integrator2/1
  Integrator2/1 -> Py/1
  Integrator3/1 -> Px/1

== system SimulationV2/ModeleNonLineaire1/ModeleNonLineaire/A2Ps1 ==
  Ax : Inport
  Ay : Inport  Port=2
  z : Inport  Port=3
  Px : Inport  Port=4
  Py : Inport  Port=5
  Add : Sum  Inputs=+-+
  Product : Product
  Product1 : Product
  Pz : Outport
  wires:
  Ax/1 -> Product/1
  Ay/1 -> Product1/1
  Px/1 -> Product1/2
  Py/1 -> Product/2
  z/1 -> Add/3
  Add/1 -> Pz/1

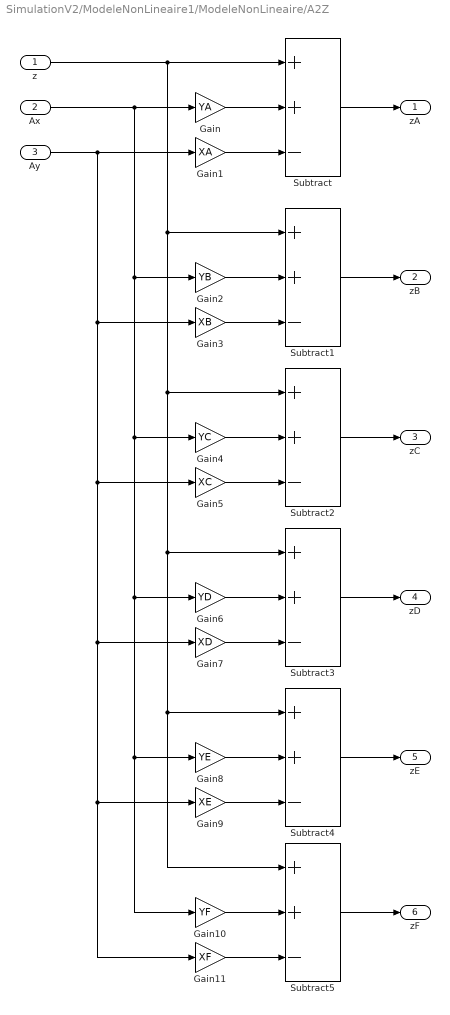
== system SimulationV2/ModeleNonLineaire1/ModeleNonLineaire/A2Z ==
  z : Inport
  Ax : Inport  Port=2
  Ay : Inport  Port=3
  Gain : Gain  Gain=YA
  Gain1 : Gain  Gain=XA
  Gain10 : Gain  Gain=YF
  Gain11 : Gain  Gain=XF
  Gain2 : Gain  Gain=YB
  Gain3 : Gain  Gain=XB
  Gain4 : Gain  Gain=YC
  Gain5 : Gain  Gain=XC
  Gain6 : Gain  Gain=YD
  Gain7 : Gain  Gain=XD
  Gain8 : Gain  Gain=YE
  Gain9 : Gain  Gain=XE
  Subtract{,1..5} (6 alike) : Sum  Inputs=++-
  zA : Outport
  zB : Outport  Port=2
  zC : Outport  Port=3
  zD : Outport  Port=4
  zE : Outport  Port=5
  zF : Outport  Port=6
  wires:
  Gain/1 -> Subtract/2
  Gain1/1 -> Subtract/3
  Subtract/1 -> zA/1
  Gain2/1 -> Subtract1/2
  Gain3/1 -> Subtract1/3
  Subtract1/1 -> zB/1
  Gain4/1 -> Subtract2/2
  Gain5/1 -> Subtract2/3
  Subtract2/1 -> zC/1
  Gain6/1 -> Subtract3/2
  Gain7/1 -> Subtract3/3
  Subtract3/1 -> zD/1
  Gain8/1 -> Subtract4/2
  Gain9/1 -> Subtract4/3
  Subtract4/1 -> zE/1
  Gain10/1 -> Subtract5/2
  Gain11/1 -> Subtract5/3
  Subtract5/1 -> zF/1
  z/1 -> Subtract5/1, Subtract4/1, Subtract3/1, Subtract2/1, Subtract1/1, Subtract/1
  Ax/1 -> Gain10/1, Gain8/1, Gain6/1, Gain4/1, Gain2/1, Gain/1
  Ay/1 -> Gain11/1, Gain9/1, Gain7/1, Gain5/1, Gain3/1, Gain1/1

== system SimulationV2/ModeleNonLineaire1/ModeleNonLineaire/F2Vz ==
  FA : Inport
  FB : Inport  Port=2
  FC : Inport  Port=3
  Add : Sum  Inputs=++++
  Constant : Constant  Value=g
  Gain : Gain  Gain=1/mtot
  Gain1 : Gain  Gain=1/mtot
  Gain2 : Gain  Gain=1/mtot
  Integrator : Integrator
  Integrator1 : Integrator  InitialCondition=Pzeq
  Vz : Outport
  z : Outport  Port=2
  wires:
  Constant/1 -> Add/1
  FA/1 -> Gain/1
  FB/1 -> Gain1/1
  FC/1 -> Gain2/1
  Gain2/1 -> Add/4
  Gain1/1 -> Add/3
  Gain/1 -> Add/2
  Add/1 -> Integrator/1
  Integrator/1 -> Integrator1/1, Vz/1
  Integrator1/1 -> z/1

== system SimulationV2/ModeleNonLineaire1/ModeleNonLineaire/F2Wx ==
  FA : Inport
  FB : Inport  Port=2
  FC : Inport  Port=3
  Py : Inport  Port=4
  Add : Sum  Inputs=++++
  Gain : Gain  Gain=YA/Jx
  Gain1 : Gain  Gain=YB/Jx
  Gain2 : Gain  Gain=YC/Jx
  Gain3 : Gain  Gain=mS*g/Jx
  Integrator : Integrator
  Integrator1 : Integrator
  Wx : Outport
  Ax : Outport  Port=2
  wires:
  FA/1 -> Gain/1
  FB/1 -> Gain1/1
  FC/1 -> Gain2/1
  Add/1 -> Integrator/1
  Integrator/1 -> Integrator1/1, Wx/1
  Py/1 -> Gain3/1
  Gain3/1 -> Add/4
  Gain2/1 -> Add/3
  Gain1/1 -> Add/2
  Gain/1 -> Add/1
  Integrator1/1 -> Ax/1

== system SimulationV2/ModeleNonLineaire1/ModeleNonLineaire/F2Wy ==
  FA : Inport
  FB : Inport  Port=2
  FC : Inport  Port=3
  Px : Inport  Port=4
  Add : Sum  Inputs=++++
  Gain : Gain  Gain=-XA/Jy
  Gain1 : Gain  Gain=-XB/Jy
  Gain2 : Gain  Gain=-XC/Jy
  Gain3 : Gain  Gain=-mS*g/Jy
  Integrator : Integrator
  Integrator1 : Integrator
  Wy : Outport
  Ay : Outport  Port=2
  wires:
  FA/1 -> Gain/1
  FB/1 -> Gain1/1
  FC/1 -> Gain2/1
  Add/1 -> Integrator/1
  Integrator/1 -> Integrator1/1, Wy/1
  Px/1 -> Gain3/1
  Gain3/1 -> Add/4
  Gain2/1 -> Add/3
  Gain1/1 -> Add/2
  Gain/1 -> Add/1
  Integrator1/1 -> Ay/1

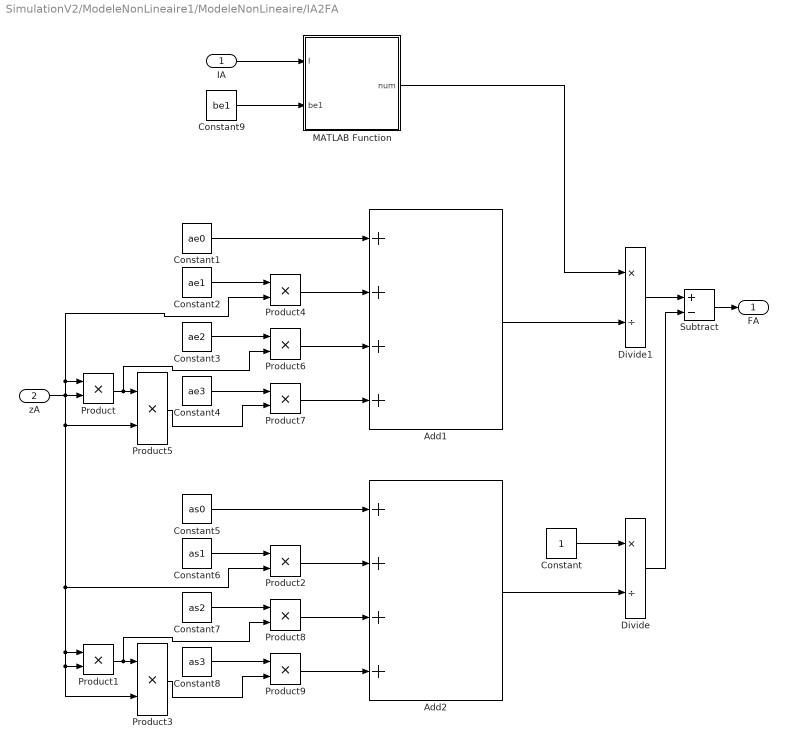
== system SimulationV2/ModeleNonLineaire1/ModeleNonLineaire/IA2FA ==
  IA : Inport
  zA : Inport  Port=2
  Add1 : Sum  Inputs=++++
  Add2 : Sum  Inputs=++++
  Constant : Constant
  Constant1 : Constant  Value=ae0
  Constant2 : Constant  Value=ae1
  Constant3 : Constant  Value=ae2
  Constant4 : Constant  Value=ae3
  Constant5 : Constant  Value=as0
  Constant6 : Constant  Value=as1
  Constant7 : Constant  Value=as2
  Constant8 : Constant  Value=as3
  Constant9 : Constant  Value=be1
  Divide : Product  Inputs=*/
  Divide1 : Product  Inputs=*/
  MATLAB Function : MATLAB Function  TreatAsAtomicUnit=on
  Product{,1..9} (10 alike) : Product
  Subtract : Sum  Inputs=+-
  FA : Outport
  wires:
  Product/1 -> Product6/2, Product5/1
  Constant1/1 -> Add1/1
  Constant2/1 -> Product4/1
  Product4/1 -> Add1/2
  Constant3/1 -> Product6/1
  Product6/1 -> Add1/3
  Constant4/1 -> Product7/1
  Product5/1 -> Product7/2
  Product7/1 -> Add1/4
  Product1/1 -> Product8/2, Product3/1
  Constant5/1 -> Add2/1
  Constant6/1 -> Product2/1
  Product2/1 -> Add2/2
  Constant7/1 -> Product8/1
  Product8/1 -> Add2/3
  Constant8/1 -> Product9/1
  Product3/1 -> Product9/2
  Product9/1 -> Add2/4
  zA/1 -> Product4/2, Product/1, Product3/2, Product1/2, Product1/1, Product2/2, Product5/2, Product/2
  Constant/1 -> Divide/1
  Add2/1 -> Divide/2
  Add1/1 -> Divide1/2
  Divide1/1 -> Subtract/1
  Subtract/1 -> FA/1
  Divide/1 -> Subtract/2
  Constant9/1 -> MATLAB Function/2(be1)
  IA/1 -> MATLAB Function/1(I)
  MATLAB Function/1(num) -> Divide1/1

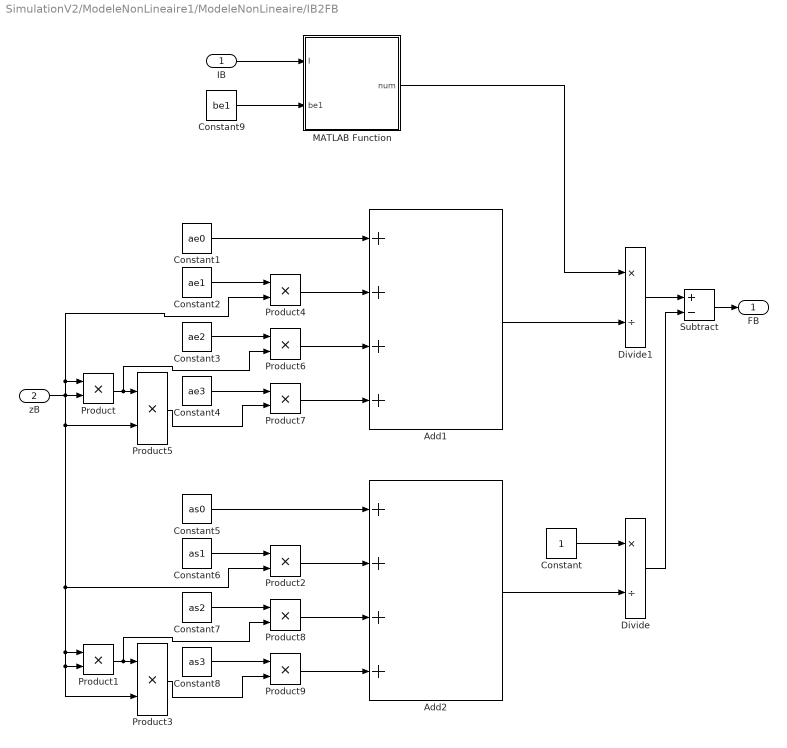
== system SimulationV2/ModeleNonLineaire1/ModeleNonLineaire/IB2FB ==
  IB : Inport
  zB : Inport  Port=2
  Add1 : Sum  Inputs=++++
  Add2 : Sum  Inputs=++++
  Constant : Constant
  Constant1 : Constant  Value=ae0
  Constant2 : Constant  Value=ae1
  Constant3 : Constant  Value=ae2
  Constant4 : Constant  Value=ae3
  Constant5 : Constant  Value=as0
  Constant6 : Constant  Value=as1
  Constant7 : Constant  Value=as2
  Constant8 : Constant  Value=as3
  Constant9 : Constant  Value=be1
  Divide : Product  Inputs=*/
  Divide1 : Product  Inputs=*/
  MATLAB Function : MATLAB Function  TreatAsAtomicUnit=on
  Product{,1..9} (10 alike) : Product
  Subtract : Sum  Inputs=+-
  FB : Outport
  wires:
  Product/1 -> Product6/2, Product5/1
  Constant1/1 -> Add1/1
  Constant2/1 -> Product4/1
  Product4/1 -> Add1/2
  Constant3/1 -> Product6/1
  Product6/1 -> Add1/3
  Constant4/1 -> Product7/1
  Product5/1 -> Product7/2
  Product7/1 -> Add1/4
  Product1/1 -> Product8/2, Product3/1
  Constant5/1 -> Add2/1
  Constant6/1 -> Product2/1
  Product2/1 -> Add2/2
  Constant7/1 -> Product8/1
  Product8/1 -> Add2/3
  Constant8/1 -> Product9/1
  Product3/1 -> Product9/2
  Product9/1 -> Add2/4
  zB/1 -> Product4/2, Product/1, Product3/2, Product1/2, Product1/1, Product2/2, Product5/2, Product/2
  Constant/1 -> Divide/1
  Add2/1 -> Divide/2
  Add1/1 -> Divide1/2
  Divide1/1 -> Subtract/1
  Subtract/1 -> FB/1
  Divide/1 -> Subtract/2
  Constant9/1 -> MATLAB Function/2(be1)
  IB/1 -> MATLAB Function/1(I)
  MATLAB Function/1(num) -> Divide1/1

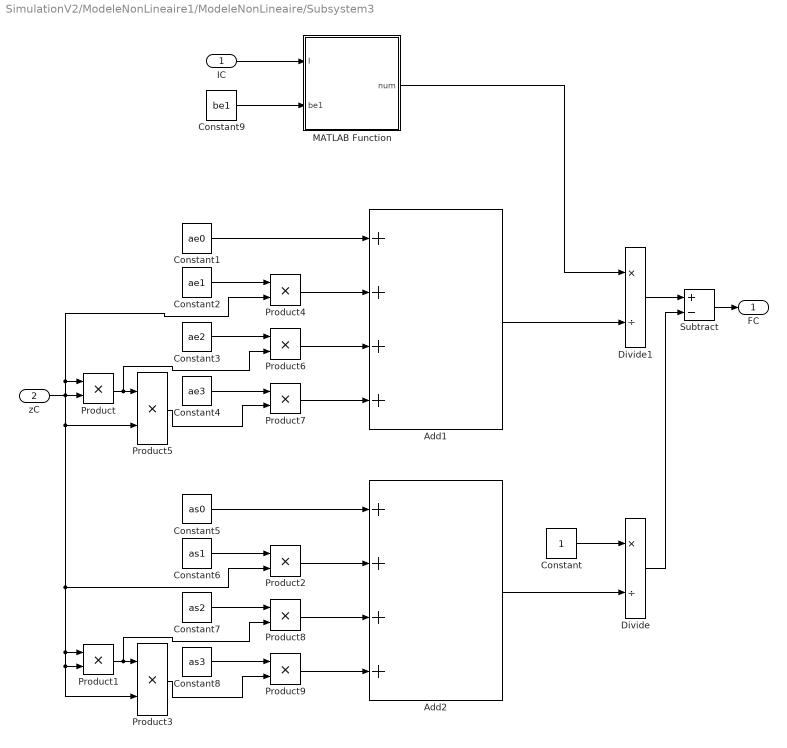
== system SimulationV2/ModeleNonLineaire1/ModeleNonLineaire/Subsystem3 ==
  IC : Inport
  zC : Inport  Port=2
  Add1 : Sum  Inputs=++++
  Add2 : Sum  Inputs=++++
  Constant : Constant
  Constant1 : Constant  Value=ae0
  Constant2 : Constant  Value=ae1
  Constant3 : Constant  Value=ae2
  Constant4 : Constant  Value=ae3
  Constant5 : Constant  Value=as0
  Constant6 : Constant  Value=as1
  Constant7 : Constant  Value=as2
  Constant8 : Constant  Value=as3
  Constant9 : Constant  Value=be1
  Divide : Product  Inputs=*/
  Divide1 : Product  Inputs=*/
  MATLAB Function : MATLAB Function  TreatAsAtomicUnit=on
  Product{,1..9} (10 alike) : Product
  Subtract : Sum  Inputs=+-
  FC : Outport
  wires:
  Product/1 -> Product6/2, Product5/1
  Constant1/1 -> Add1/1
  Constant2/1 -> Product4/1
  Product4/1 -> Add1/2
  Constant3/1 -> Product6/1
  Product6/1 -> Add1/3
  Constant4/1 -> Product7/1
  Product5/1 -> Product7/2
  Product7/1 -> Add1/4
  Product1/1 -> Product8/2, Product3/1
  Constant5/1 -> Add2/1
  Constant6/1 -> Product2/1
  Product2/1 -> Add2/2
  Constant7/1 -> Product8/1
  Product8/1 -> Add2/3
  Constant8/1 -> Product9/1
  Product3/1 -> Product9/2
  Product9/1 -> Add2/4
  zC/1 -> Product4/2, Product/1, Product3/2, Product1/2, Product1/1, Product2/2, Product5/2, Product/2
  Constant/1 -> Divide/1
  Add2/1 -> Divide/2
  Add1/1 -> Divide1/2
  Divide1/1 -> Subtract/1
  Subtract/1 -> FC/1
  Divide/1 -> Subtract/2
  Constant9/1 -> MATLAB Function/2(be1)
  IC/1 -> MATLAB Function/1(I)
  MATLAB Function/1(num) -> Divide1/1

== system SimulationV2/ModeleNonLineaire1/ModeleNonLineaire/VA2IA ==
  In1 : Inport
  Gain : Gain  Gain=1/LA
  Gain1 : Gain  Gain=RA/LA
  Integrator : Integrator  InitialCondition=-0.496058088227384
  Subtract : Sum  Inputs=+-
  Out1 : Outport
  wires:
  In1/1 -> Gain/1
  Integrator/1 -> Out1/1, Gain1/1
  Subtract/1 -> Integrator/1
  Gain/1 -> Subtract/1
  Gain1/1 -> Subtract/2

== system SimulationV2/ModeleNonLineaire1/ModeleNonLineaire/VB2IB ==
  In1 : Inport
  Gain : Gain  Gain=1/LB
  Gain1 : Gain  Gain=RB/LB
  Integrator : Integrator  InitialCondition=-0.496058088227384
  Subtract : Sum  Inputs=+-
  Out1 : Outport
  wires:
  In1/1 -> Gain/1
  Integrator/1 -> Out1/1, Gain1/1
  Subtract/1 -> Integrator/1
  Gain/1 -> Subtract/1
  Gain1/1 -> Subtract/2

== system SimulationV2/ModeleNonLineaire1/ModeleNonLineaire/VC2IC ==
  In1 : Inport
  Gain : Gain  Gain=1/LC
  Gain1 : Gain  Gain=RC/LC
  Integrator : Integrator  InitialCondition=-0.496058088227384
  Subtract : Sum  Inputs=+-
  Out1 : Outport
  wires:
  In1/1 -> Gain/1
  Integrator/1 -> Out1/1, Gain1/1
  Subtract/1 -> Integrator/1
  Gain/1 -> Subtract/1
  Gain1/1 -> Subtract/2

== matlab function SimulationV2/ModeleNonLineaire1/ModeleNonLineaire/IB2FB/MATLAB Function ==
  data: I input; num output; be1 input
function num = fcn(I,be1)
%#codegen

num = (I^2+be1*abs(I))*sign(I);

== matlab function SimulationV2/ModeleNonLineaire1/ModeleNonLineaire/IA2FA/MATLAB Function ==
  data: I input; num output; be1 input
function num = fcn(I,be1)
%#codegen

num = (I^2+be1*abs(I))*sign(I);

== matlab function SimulationV2/ModeleNonLineaire1/ModeleNonLineaire/Subsystem3/MATLAB Function ==
  data: I input; num output; be1 input
function num = fcn(I,be1)
%#codegen

num = (I^2+be1*abs(I))*sign(I);
